simulink library "FeaturePath"  (R2022b)
settings: Solver=VariableStepAuto  StartTime=0.0  StopTime=10.0  RelTol=1e-3
undefined symbols (not defined in the file or in its folder): AddSimEventList, groupNumber, groupPath, ok, partitionNumber, RtcRequestListHash
libraries: HandyTextFile x7, $bdroot x1
settings Model: Creator=kl13806  LastModifiedBy=kl13806
settings SolverCC: AlgebraicLoopSolver=TrustRegion
settings DebuggingCC: UnconnectedInputMsg=warning  UnconnectedOutputMsg=warning  UnconnectedLineMsg=warning  SFMachineParentedDataDiag=warning  ArithmeticOperatorsInVariantConditions=warning
settings ModelReferenceCC: EnableRefExpFcnMdlSchedulingChecks=on
settings SFSimCC: SimUseLocalCustomCode=off  CustomCodeUndefinedFunction=UseInterfaceOnly
settings RTWCC: TLCOptions=-aINCLUDE_ASYNCH_CONSOLE=1  RTWUseLocalCustomCode=off  DLArmComputeVersion=19.05
settings CodeAppCC: StateflowObjectComments=on

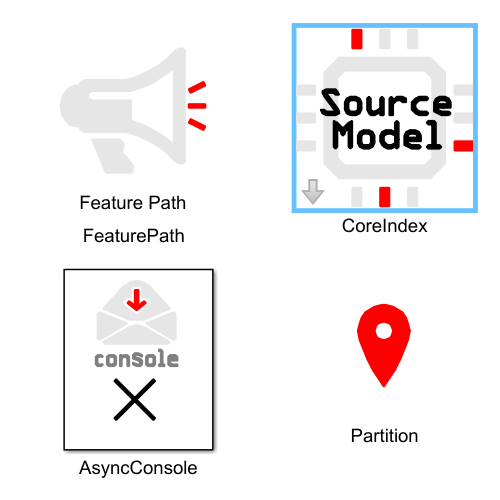
[thumbnail: Simulink's stored preview of the top-level diagram]
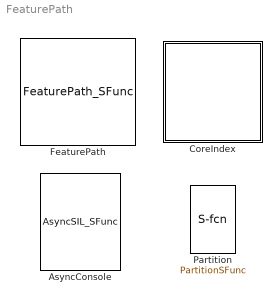
== system FeaturePath ==
  AsyncConsole : M-S-Function  FunctionName=AsyncSIL_SFunc  Parameters=AddSimEventList,RtcRequestListHash,AsyncWakeMsec  mask(Talaria Async Target Console){Option=Disable async-console code, AsyncWakeMsec=2}
      mask prompts: Option "Code generation behavior:"; AsyncWakeMsec "Windows thread millisecond wake rate:"
      mask help: This block is a cheat to set the TLCOptions in a model's configuration parameters to control the generation of code for asynchronous console parsing. When the block is initialized in diagram updates, it updates TLCOptions appropriately. This means when this block is deleted, is stops updating TLCOptions. To disable the async code, uncheck boxes and update diagram before removing this block!
      mask init:
      | [AddSimEventList,RtcRequestListHash] = AsyncConsoleMask.DoInit(gcbh,Option);
      mask Callback Option: AsyncConsoleMask.CB_Option(gcbh);
      mask Display:
      | % retrieve icon definition
      | [path,w,h] = AsyncConsoleMask.Icon(Option);
      | 
      | % retrieve the block's pixel size
      | pos = get(gcbh,'position');
      | bw = pos(3) - pos(1);
      | bh = pos(4) - pos(2);
      | 
      | % draw centered icon
      | xAdj = bw/2 - w/2;
      | yAdj = bh/2 - h/2;
      | for i=1:length(path)
      | 	patch(path(i).x+xAdj, path(i).y+yAdj, path(i).rgb);
      | end
  CoreIndex : Subsystem  mask(Talaria Core Index){Role=Source Model, CoreIndex=8, Config=[], AddressingMode=Directly include core number in message identifiers (i.e. simple and static), CrossCoreApi=FourListChipManager, CrossCoreAllocation=LocalCore, CrossCoreSampleTime=-1, BasePeriod=[], TriggerInit=[185 -1 280 96]}
      mask prompts: Role "Role of model in the system"; Config "CoreIndexConfig"; AddressingMode "Multi-core Token Addressing Mode"; CrossCoreApi "Interface Type"; CrossCoreAllocation "Buffer Allocation"; CrossCoreSampleTime "Cross-core sample time (-1 for automatic):"; BasePeriod "System Base Period in Seconds:"; TriggerInit "Hidden: dialog open, MoveFcn"
      mask help: This block specifies the role of this model in the system. It impacts the behavior of all feature blocks.
      mask init:
      | blkh=gcbh;
      | BeforeAssert=Config;
      | Config=BTConfig.Assert(blkh,Config);
      | [ok,Config] = CoreIndexMask.DoInit(gcbh,Role,Config,BeforeAssert);
      | Config.Validate();
      | Config.DoMaskInit(blkh);
      settings: MoveFcn=CoreIndexMask.CB_TriggerInit(gcbh);
      mask TypeOptions Role: Processor Core 0 | Processor Core 1 | Processor Core 2 | Processor Core 3 | Processor Core 4 | Processor Core 5 | Processor Core 6 | Processor Core 7 | Source Model | Translation Engine | Interpretation Engine
      mask Callback Config: CoreIndexMask.CB_Config(gcbh);
      mask TypeOptions AddressingMode: Indirect core determination via table lookup (i.e. use Partition blocks) | Directly include core number in message identifiers (i.e. simple and static)
      mask TypeOptions CrossCoreApi: None | FourList | FourListChipManager
      mask Callback CrossCoreApi: CoreIndexMask.CB_CrossCoreApi(gcbh);
      mask TypeOptions CrossCoreAllocation: None | LocalCore | AllLocalChip
      mask Callback TriggerInit: CoreIndexMask.CB_TriggerInit(gcbh);
      mask DialogControl SystemGroup Prompt: System Cross-Chip Communications
      mask DialogControl PeriodGroup Prompt: Multi-core Shared Time Base
      mask DialogControl ErrorContainer Prompt: Error Messages
      mask Display:
      | % retrieve icon definition
      | [path,w,h] = CoreIndexMask.Icon(gcbh);
      | 
      | % retrieve the block's pixel size
      | pos = get(gcbh,'position');
      | bw = pos(3) - pos(1);
      | bh = pos(4) - pos(2);
      | 
      | % draw centered icon
      | xAdj = bw/2 - w/2;
      | yAdj = bh/2 - h/2;
      | for i=1:length(path)
      | 	patch(path(i).x+xAdj, path(i).y+yAdj, path(i).rgb);
      | end
      | 
      | % show the name or an X
      | if (exist('ok','var') && ok)
      | 	patch(0,0,[1 1 1]);
      | 	patch(bw,bh,[1 1 1]);
      | else
      | 	tx=bw*0.03;
      | 	ty=bh*0.03;
      | 	patch([0 tx bw bw-tx], [ty 0 bh-ty bh], [1 0 0]);
      | 	patch([0 bw-tx bw tx], [bh-ty 0 ty bh], [1 0 0]);
      | end
  FeaturePath : M-S-Function  FunctionName=FeaturePath_SFunc  mask(Talaria Feature Path){FeatureName=, IsGroup=off, GroupNumber=-1, IsModule=off, TriggerInit=[40 -6 155 101]}
      mask prompts: FeatureName "Feature path name:"; IsGroup "Declare an overlay group"; GroupNumber "Group number:"; IsModule "Declare a module at this path level"; TriggerInit "Hidden: dialog open, MoveFcn"
      mask help: This block impacts the external name of all Talaria configuration blocks (e.g. RTC, TOP, TuneVar, TSP, etc) found in the same subsystem and below in Simulink's subsystem hierarchy. Also this block optionally declares a module at this level of the feature path to assist with external integration.
      mask init:
      | [ok,fullPath,groupNumber] = FeaturePathMask.DoInit(gcbh,FeatureName,IsGroup,GroupNumber);
      settings: MoveFcn=FeaturePathMask.CB_TriggerInit(gcbh);
      mask Help:
      | The Talaria configuration blocks such as Runtime Control (RTC) and Tune Variable (TuneVar) rely on FeaturePath blocks to determine their unique name in a model. Each FeaturePath block specifies a piece of an overall name much like each folder in a filesystem is a piece of a file's complete path.
      | 
      | In addition to the "path" responsibility, the FeaturePath block also has the following optional roles it can serve:
      | 
      | <b>Overlay Group</b>: When this role is enabled for a FeaturePath block it specifies that the block sits at the top of a feature large enough to define it own type of room mode. All of the target overlay parameters (TOPs) found within this overlay group will together comprise a complete set of overlay data for the feature. Note that overlay groups cannot be nested. Once a FeaturePath block specifies that it defines an overlay group, any FeaturePath blocks below it in the Simulink subsystem hierarchy will not be able to define its own group.
      | 
      | <b>Declare Module</b>: With this role enabled, a FeaturePath block indicates to external systems that feature objects (e.g. TuneVars, TOPs, TSPs, RTCs) found below it are logically grouped together as a "module". This specification does not impact code or behavior, but is just an exported specification (e.g. XML) to assist with integration. Note that FeaturePath blocks must already be within an overlay group to successfully declare themselves as a module. This limitation is because Talaria does not support modules that include multiple overlay groups within them. Also take note that the highest level FeaturePath module may serve additional roles in the tuning infrastructure and/or control logic system such as providing the filename for tuning files or a shared classname for control logic systems.
      mask Callback IsGroup: FeaturePathMask.CB_IsGroup(gcbh);
      mask Callback TriggerInit: FeaturePathMask.CB_TriggerInit(gcbh);
      mask DialogControl ParameterGroupVar Prompt: Feature Name
      mask DialogControl OverlayGroupVar Prompt: Overlay Group Settings
      mask DialogControl ButtonFindGroupNumber Prompt: Find unused number
      mask DialogControl ButtonFindGroupNumber Callback: FeaturePathMask.CB_FindFreeNumber(gcbh);
      mask DialogControl ModuleGroupVar Prompt: Module Settings
      mask DialogControl AutomationGroupVar Prompt: Automation
      mask DialogControl PromoteMe Prompt: Promote feature-path name to parent mask
      mask DialogControl PromoteMe Callback: FeaturePathMask.CB_PromoteMe(gcbh)
      mask DialogControl ErrorContainer Prompt: Error Messages
      mask Display:
      | % retrieve icon definition
      | [path,w,h] = FeaturePathMask.Icon();
      | 
      | % retrieve the block's pixel size
      | pos = get(gcbh,'position');
      | bw = pos(3) - pos(1);
      | bh = pos(4) - pos(2);
      | 
      | % draw centered icon
      | xAdj = bw/2 - w/2 - 1;
      | yAdj = bh/2 - h/2 + 4;
      | for i=1:length(path)
      |    patch(path(i).x+xAdj, path(i).y+yAdj, path(i).rgb);
      | end
      | 
      | % show the name or an X
      | if (exist('ok','var') && ok)
      |    text(bw*0.5, bh*0.08, fullPath, 'horizontalAlignment','center');
      |    if (groupNumber ~= -1)
      |       text(bw*0.5+12,bh*0.5+5,num2str(groupNumber),'horizontalAlignment','center');
      |    end
      |    patch(0,0,[1 1 1]);
      |    patch(bw,bh,[1 1 1]);
      | else
      |    tx=bw*0.03;
      |    ty=bh*0.03;
      |    patch([0 tx bw bw-tx], [ty 0 bh-ty bh], [1 0 0]);
      |    patch([0 bw-tx bw tx], [bh-ty 0 ty bh], [1 0 0]);
      | end
  Partition : M-S-Function  FunctionName=PartitionSFunc  Parameters=ok,partitionNumber,groupNumber,groupPath  mask(Talaria Partition){PartitionNumber=-1, TriggerInit=[]}
      mask prompts: PartitionNumber "Partition Number:"; TriggerInit "Hidden: dialog open, MoveFcn"
      mask help: This block defines an addressable partition of feature logic for the purposes of multi-core asymmetric multi-processing. Each overlay group supports multiple partitions comprising it each of which can be assigned to an arbitrary processor core. The use of this block located just inside a top-level atomic enables configuration blocks like RTCs and TOPs to acquire an unchanging locator ID that stays the same regardless of which processor core is eventually used to contain the logic.
      mask init:
      | [ok,partitionNumber,groupNumber,groupPath] = PartitionMask.DoInit(gcbh,PartitionNumber);
      settings: MoveFcn=PartitionMask.CB_TriggerInit(gcbh);
      mask Help: The Talaria configuration blocks such as Runtime Control (RTC) and Tune Variable (TuneVar) rely on their containing Partition block and Overlay Group to determine a processor-core independent unique ID in the system.
      mask Callback TriggerInit: PartitionMask.CB_TriggerInit(gcbh);
      mask DialogControl ButtonFindFreeNumber Prompt: Find unused number
      mask DialogControl ButtonFindFreeNumber Callback: PartitionMask.CB_FindFreeNumber(gcbh);
      mask DialogControl ErrorContainer Prompt: Error Messages
      mask Display:
      | % retrieve icon definition
      | [path,w,h] = PartitionMask.Icon(partitionNumber);
      | 
      | % retrieve the block's pixel size
      | pos = get(gcbh,'position');
      | bw = pos(3) - pos(1);
      | bh = pos(4) - pos(2);
      | 
      | % draw centered icon
      | xAdj = bw/2 - w/2;
      | yAdj = bh/2 - h/2 + 4;
      | for i=1:length(path)
      | 	patch(path(i).x+xAdj, path(i).y+yAdj, path(i).rgb);
      | end
      | 
      | % show the name or an X
      | if (exist('ok','var') && ok)
      | 	text(bw*0.5, bh*0.1, num2str(partitionNumber), 'horizontalAlignment','center');
      | 	patch(0,0,[1 1 1]);
      | 	patch(bw,bh,[1 1 1]);
      | else
      | 	tx=bw*0.03;
      | 	ty=bh*0.03;
      | 	patch([0 tx bw bw-tx], [ty 0 bh-ty bh], [1 0 0]);
      | 	patch([0 bw-tx bw tx], [bh-ty 0 ty bh], [1 0 0]);
      | end

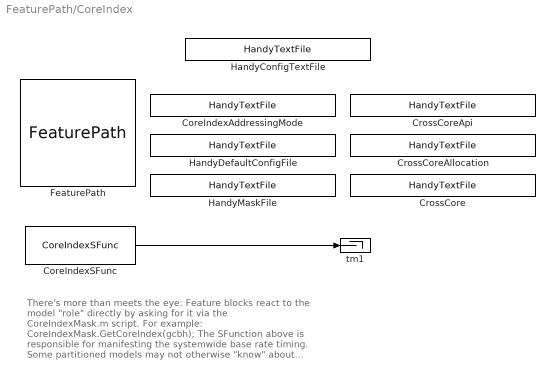
== system FeaturePath/CoreIndex ==
  note: There's more than meets the eye:
      | Feature blocks react to the model "role" directly by
      | asking for it via the CoreIndexMask.m script.
      | For example:
      | CoreIndexMask.GetCoreIndex(gcbh);
      |
      | The SFunction above is responsible for manifesting the
      | systemwide base rate timing. Some partitioned models
      | may not otherwise "know" about this rate.
  CoreIndexAddressingMode : HandyTextFile/HandyTextFile  TemplateSource=Enum  FileSuffix=Init  OpenDialogOnLoad=off  UseThisBlockName=on  AddGrandParentNamePrefix=off  TheDefaultText=|  ShowInLibBrowser=on
      | % $(FILENAME) Setup model parameters for each "Init" callback (e.g. update diagram)
      | sample_rate_in_hertz = 44100;
      | frame_size = 32;
      | sysin_channel_count = 2;
      settings: SourceProductName=Bose Talaria
  CoreIndexSFunc : M-S-Function  FunctionName=CoreIndexSFunc  Parameters=BasePeriod
  CrossCore : HandyTextFile/HandyTextFile  TemplateSource=Config  FileSuffix=Init  OpenDialogOnLoad=off  UseThisBlockName=on  AddGrandParentNamePrefix=off  TheDefaultText=|  ShowInLibBrowser=on
      | % $(FILENAME) Setup model parameters for each "Init" callback (e.g. update diagram)
      | sample_rate_in_hertz = 44100;
      | frame_size = 32;
      | sysin_channel_count = 2;
      settings: SourceProductName=Bose Talaria
  CrossCoreAllocation : HandyTextFile/HandyTextFile  TemplateSource=Enum  FileSuffix=Init  OpenDialogOnLoad=off  UseThisBlockName=on  AddGrandParentNamePrefix=off  TheDefaultText=|  ShowInLibBrowser=on
      | % $(FILENAME) Setup model parameters for each "Init" callback (e.g. update diagram)
      | sample_rate_in_hertz = 44100;
      | frame_size = 32;
      | sysin_channel_count = 2;
      settings: SourceProductName=Bose Talaria
  CrossCoreApi : HandyTextFile/HandyTextFile  TemplateSource=Enum  FileSuffix=Init  OpenDialogOnLoad=off  UseThisBlockName=on  AddGrandParentNamePrefix=off  TheDefaultText=|  ShowInLibBrowser=on
      | % $(FILENAME) Setup model parameters for each "Init" callback (e.g. update diagram)
      | sample_rate_in_hertz = 44100;
      | frame_size = 32;
      | sysin_channel_count = 2;
      settings: SourceProductName=Bose Talaria
  FeaturePath : $bdroot/FeaturePath  FeatureName=CoreIndexRole  IsGroup=off  GroupNumber=-1  IsModule=off  TriggerInit=[]
  HandyConfigTextFile : HandyTextFile/HandyTextFile  TemplateSource=Config  FileSuffix=File  OpenDialogOnLoad=off  UseThisBlockName=off  AddGrandParentNamePrefix=off  TheDefaultText=% $(FILENAME) $(PREFIX) $(SUFFIX)  ShowInLibBrowser=on
      settings: SourceProductName=Bose Talaria
  HandyDefaultConfigFile : HandyTextFile/HandyTextFile  TemplateSource=Config  FileSuffix=Init  OpenDialogOnLoad=off  UseThisBlockName=off  AddGrandParentNamePrefix=off  TheDefaultText=|  ShowInLibBrowser=on
      | % $(FILENAME) Setup model parameters for each "Init" callback (e.g. update diagram)
      | sample_rate_in_hertz = 44100;
      | frame_size = 32;
      | sysin_channel_count = 2;
      settings: SourceProductName=Bose Talaria
  HandyMaskFile : HandyTextFile/HandyTextFile  TemplateSource=<dialog fields>  FileSuffix=Mask  OpenDialogOnLoad=off  UseThisBlockName=off  AddGrandParentNamePrefix=off  TheDefaultText=|  ShowInLibBrowser=on
      | % $(FILENAME) Setup model parameters for each "Init" callback (e.g. update diagram)
      | sample_rate_in_hertz = 44100;
      | frame_size = 32;
      | sysin_channel_count = 2;
      settings: SourceProductName=Bose Talaria
  tm1 : Terminator
  wires:
  CoreIndexSFunc/1 -> tm1/1
